simulink model "SWC_HALOUT_type"  (R2021b)
settings: Solver=FixedStepDiscrete  StartTime=0.0  StopTime=10.0  FixedStep=0.001  RelTol=1e-3
values from neighbouring files (symbols this model uses):
  DIDLen_APPPedalZP = uint16(3)    [vcu_local_hdr.m]
  DIDLen_APSFunConfig = uint16(16)    [vcu_local_hdr.m]
  DIDLen_AutoLock = uint16(1)    [vcu_local_hdr.m]
  DIDLen_AutoWipHSpdEN = uint16(1)    [vcu_local_hdr.m]
  DIDLen_DKCKey = uint16(8)    [vcu_local_hdr.m]
  DIDLen_DRLDis = uint16(1)    [vcu_local_hdr.m]
  DIDLen_DynoMode = uint16(1)    [vcu_local_hdr.m]
  DIDLen_FMHTimer = uint16(1)    [vcu_local_hdr.m]
  DIDLen_LFLowPresThre = uint16(1)    [vcu_local_hdr.m]
  DIDLen_LFSensorID = uint16(4)    [vcu_local_hdr.m]
  DIDLen_LRLowPresThre = uint16(1)    [vcu_local_hdr.m]
  DIDLen_LRSensorID = uint16(4)    [vcu_local_hdr.m]
  DIDLen_NVMPedalZP = uint16(3)    [vcu_local_hdr.m]
  DIDLen_RFLowPresThre = uint16(1)    [vcu_local_hdr.m]
  DIDLen_RFSensorID = uint16(4)    [vcu_local_hdr.m]
  DIDLen_RRLowPresThre = uint16(1)    [vcu_local_hdr.m]
  DIDLen_RRSensorID = uint16(4)    [vcu_local_hdr.m]
  DIDLen_SensorMode = uint16(1)    [vcu_local_hdr.m]
  DIDLen_TireSize = uint16(16)    [vcu_local_hdr.m]
  DIDLen_TPMSLearnSta = uint16(1)    [vcu_local_hdr.m]
  DIDLen_TurnLampFLThreCurr = uint16(1)    [vcu_local_hdr.m]
  DIDLen_TurnLampFRThreCurr = uint16(1)    [vcu_local_hdr.m]
  DIDLen_TurnLampRLThreCurr = uint16(1)    [vcu_local_hdr.m]
  DIDLen_TurnLampRRThreCurr = uint16(1)    [vcu_local_hdr.m]
  DIDLen_USSConfig = uint16(16)    [vcu_local_hdr.m]
  DIDLen_WhlPres = uint16(4)    [vcu_local_hdr.m]
  DIDLen_WhlSensorBattSta = uint16(1)    [vcu_local_hdr.m]
  DIDLen_WhlTmp = uint16(4)    [vcu_local_hdr.m]
  DIDLen_WipRLSCmdCutFilter = uint16(1)    [vcu_local_hdr.m]
  DIDLen_WipRLSCmdHoldFilter = uint16(1)    [vcu_local_hdr.m]
  DIDLen_XWDMode = uint16(1)    [vcu_local_hdr.m]
  DIDNum_APPPedalZP = uint16(0x0206)    [vcu_local_hdr.m]
  DIDNum_APSFunConfig = uint16(0x0903)    [vcu_local_hdr.m]
  DIDNum_AutoLock = uint16(0x0306)    [vcu_local_hdr.m]
  DIDNum_AutoWipHSpdEN = uint16(0x0308)    [vcu_local_hdr.m]
  DIDNum_DKCKey = uint16(0x0202)    [vcu_local_hdr.m]
  DIDNum_DRLDis = uint16(0x0307)    [vcu_local_hdr.m]
  DIDNum_DynoMode = uint16(0x0203)    [vcu_local_hdr.m]
  DIDNum_FMHTimer = uint16(0x0305)    [vcu_local_hdr.m]
  DIDNum_LFLowPresThre = uint16(0x0B08)    [vcu_local_hdr.m]
  DIDNum_LFSensorID = uint16(0x0B01)    [vcu_local_hdr.m]
  DIDNum_LRLowPresThre = uint16(0x0B0A)    [vcu_local_hdr.m]
  DIDNum_LRSensorID = uint16(0x0B03)    [vcu_local_hdr.m]
  DIDNum_NVMPedalZP = uint16(0x0207)    [vcu_local_hdr.m]
  DIDNum_RFLowPresThre = uint16(0x0B09)    [vcu_local_hdr.m]
  DIDNum_RFSensorID = uint16(0x0B02)    [vcu_local_hdr.m]
  DIDNum_RRLowPresThre = uint16(0x0B0B)    [vcu_local_hdr.m]
  DIDNum_RRSensorID = uint16(0x0B04)    [vcu_local_hdr.m]
  DIDNum_SensorMode = uint16(0x0B0C)    [vcu_local_hdr.m]
  DIDNum_TireSize = uint16(0x0902)    [vcu_local_hdr.m]
  DIDNum_TPMSLearnSta = uint16(0x0B0D)    [vcu_local_hdr.m]
  DIDNum_TurnLampFLThreCurr = uint16(0x0303)    [vcu_local_hdr.m]
  DIDNum_TurnLampFRThreCurr = uint16(0x0301)    [vcu_local_hdr.m]
  DIDNum_TurnLampRLThreCurr = uint16(0x0304)    [vcu_local_hdr.m]
  DIDNum_TurnLampRRThreCurr = uint16(0x0302)    [vcu_local_hdr.m]
  DIDNum_USSConfig = uint16(0x0901)    [vcu_local_hdr.m]
  DIDNum_WhlPres = uint16(0x0B05)    [vcu_local_hdr.m]
  DIDNum_WhlSensorBattSta = uint16(0x0B07)    [vcu_local_hdr.m]
  DIDNum_WhlTmp = uint16(0x0B06)    [vcu_local_hdr.m]
  DIDNum_WipRLSCmdCutFilter = uint16(0x030A)    [vcu_local_hdr.m]
  DIDNum_WipRLSCmdHoldFilter = uint16(0x0309)    [vcu_local_hdr.m]
  DIDNum_XWDMode = uint16(0x0201)    [vcu_local_hdr.m]
  ENUM_TPMSLearnStatus_LEARNED = uint8(  1  )    [vcu_local_hdr.m]
  ENUM_TPMSLearnStatus_LEARNFAIL = uint8(  2  )    [vcu_local_hdr.m]
  ENUM_TPMSLearnStatus_NOTLEARN = uint8(  0  )    [vcu_local_hdr.m]
  FALSE = boolean( 0 )    [vcu_local_hdr.m]    (also in vcu_local_hdrTA2.m)
  TRUE = boolean( 1 )    [vcu_local_hdr.m]    (also in vcu_local_hdrTA2.m)
  ZERO_INT = uint8(0)    [vcu_local_hdr.m]    (also in vcu_local_hdrTA2.m)
undefined symbols (not defined in the file or in its folder): f32_ApsOutVehSpdSig, R_DIDWriteCDD_CSOP_DIDSet_APPPedalZP, R_DIDWriteCDD_CSOP_DIDSet_APSFunConfig, R_DIDWriteCDD_CSOP_DIDSet_AutoLock, R_DIDWriteCDD_CSOP_DIDSet_AutoWipHSpdEN, R_DIDWriteCDD_CSOP_DIDSet_DKCKey, R_DIDWriteCDD_CSOP_DIDSet_DRLDis, R_DIDWriteCDD_CSOP_DIDSet_DynoMode, R_DIDWriteCDD_CSOP_DIDSet_FMHTimer, R_DIDWriteCDD_CSOP_DIDSet_LFLowPresThre, R_DIDWriteCDD_CSOP_DIDSet_LFSensorID, R_DIDWriteCDD_CSOP_DIDSet_LRLowPresThre, R_DIDWriteCDD_CSOP_DIDSet_LRSensorID, R_DIDWriteCDD_CSOP_DIDSet_NVMPedalZP, R_DIDWriteCDD_CSOP_DIDSet_RFLowPresThre, R_DIDWriteCDD_CSOP_DIDSet_RFSensorID, R_DIDWriteCDD_CSOP_DIDSet_RRLowPresThre, R_DIDWriteCDD_CSOP_DIDSet_RRSensorID, R_DIDWriteCDD_CSOP_DIDSet_SensorMode, R_DIDWriteCDD_CSOP_DIDSet_TireSize, R_DIDWriteCDD_CSOP_DIDSet_TPMSLearnSta, R_DIDWriteCDD_CSOP_DIDSet_TurnLampFLThreCurr, R_DIDWriteCDD_CSOP_DIDSet_TurnLampFRThreCurr, R_DIDWriteCDD_CSOP_DIDSet_TurnLampRLThreCurr, R_DIDWriteCDD_CSOP_DIDSet_TurnLampRRThreCurr, R_DIDWriteCDD_CSOP_DIDSet_USSConfig, R_DIDWriteCDD_CSOP_DIDSet_WhlPres, R_DIDWriteCDD_CSOP_DIDSet_WhlSensorBattSta, R_DIDWriteCDD_CSOP_DIDSet_WhlTmp, R_DIDWriteCDD_CSOP_DIDSet_WipRLSCmdCutFilter, R_DIDWriteCDD_CSOP_DIDSet_WipRLSCmdHoldFilter, R_DIDWriteCDD_CSOP_DIDSet_XWDMode, R_FDCCDD_Inner_CSOP_FDC_AppCallSleep, R_HALINCDD_CSOP_PAS_Handler, R_HALINCDD_CSOP_UDS_Main, R_HALOUT_APS_CSOP_ApsOutput, R_HALOUTCDD_CSOP_AppNmStateReq, R_HALOUTCDD_CSOP_ResetPedalZeroPosDone, R_HALOUTCDD_CSOP_SetAcoreRebootCmdACK, R_HALOUTCDD_CSOP_SetHazardIND, R_HALOUTCDD_CSOP_SetSysPwrStat, R_HALOUTCDD_CSOP_SleepRequest, R_HALOUTCDD_CSOP_TPMSSensorIDRegSetResults, R_IOExpOUT_CDD_CSOP_IOExpSetVal, R_J1939_CAN1_FD1_CE100_0_CSOP_Write_CAN1_FD1_CE100_0, R_J1939_CAN1_FD1_CE100_1_CSOP_Write_CAN1_FD1_CE100_1, R_NVMWriteCDD_Inner_NVM_WriteOperation, R_UDSCDD_CSOP_DdmRestartOperationCycle, R_WDGCDD_CSOP_Call_WDG_AppEnd, u16_DIDLen_APPPedalZP, u16_DIDLen_APSFunConfig, u16_DIDLen_AutoLock, u16_DIDLen_AutoWipHSpdEN, u16_DIDLen_DKCKey, u16_DIDLen_DRLDis, u16_DIDLen_DynoMode, u16_DIDLen_FMHTimer, u16_DIDLen_LFLowPresThre, u16_DIDLen_LFSensorID, u16_DIDLen_LRLowPresThre ... (+95)
libraries: FVT_lib x142, simulink x107, hdlsllib x6, hcu_lib x5, halout x1
(part 8 of 8)

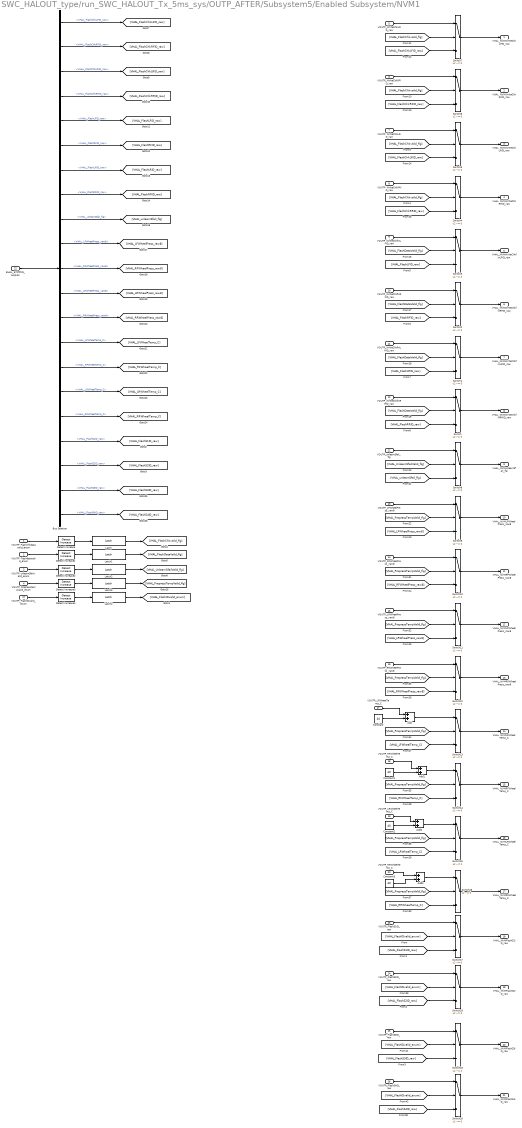
== system SWC_HALOUT_type/run_SWC_HALOUT_Tx_5ms_sys/OUTP_AFTER/Subsystem5/Enabled Subsystem/NVM1 ==
  VOUTP_Flashchkdatavalid_enum : Inport
  VOUTP_Flashdatavalid_enum : Inport  Port=2
  VOUTP_unlearnSfailvalid_enum : Inport  Port=3
  VOUTP_Prepresstempvalid_enum : Inport  Port=4
  VOUTP_WriteChkLFID_raw : Inport  Port=5
  VOUTP_WriteChkRFID_raw : Inport  Port=6
  VOUTP_WriteChkLRID_raw : Inport  Port=7
  VOUTP_WriteChkRRID_raw : Inport  Port=8
  VOUTP_WriteChkfinLFID_raw : Inport  Port=9
  VOUTP_WriteChkfinRFID_raw : Inport  Port=10
  VOUTP_WriteChkfinLRID_raw : Inport  Port=11
  VOUTP_WriteChkfinRRID_raw : Inport  Port=12
  VOUTP_LFWheelPress_raw8 : Inport  Port=13
  VOUTP_RFWheelPress_raw8 : Inport  Port=14
  VOUTP_LRWheelPress_raw8 : Inport  Port=15
  VOUTP_RRWheelPress_raw8 : Inport  Port=16
  VOUTP_LFWheelTemp_C : Inport  Port=17
  VOUTP_RFWheelTemp_C : Inport  Port=18
  VOUTP_LRWheelTemp_C : Inport  Port=19
  VOUTP_RRWheelTemp_C : Inport  Port=20
  VOUTP_unlearnSfali_flg : Inport  Port=21
  BHAL_SYSTPMS_outputs : Inport  Port=22
  VOUTP_FlashS1ID_raw : Inport  Port=23
  VOUTP_FlashS2ID_raw : Inport  Port=24
  VOUTP_FlashS3ID_raw : Inport  Port=25
  VOUTP_FlashS4ID_raw : Inport  Port=26
  VOUTP_FlashIDvalid_enum : Inport  Port=27
  Add{,1..3} (4 alike) : Sum
  Bus Selector : BusSelector  OutputSignals=VHAL_FlashChkLFID_raw,VHAL_FlashChkRFID_raw,VHAL_FlashChkLRID_raw,VHAL_FlashChkRRID_raw,VHAL_FlashLFID_raw,VHAL_FlashRFID_raw,VHAL_FlashLRID_raw,VHAL_FlashRRID_raw,VHAL_unlearnSfali_flg,VHAL_LFWheelPress_raw8,VHAL_RFWheelPress_raw8,VHAL_LRWheelPress_raw8,VHAL_RRWheelPress_raw8,VHAL_LFWheelTemp_C,VHAL_RFWheelTemp_C,VHAL_LRWheelTemp_C,VHAL_RRWheelTemp_C,VHAL_FlashS1ID_raw,VHAL_FlashS2ID_raw,VHAL_FlashS3ID_raw,VHAL_FlashS4ID_raw
  Constant{,1..3} (4 alike) : Constant  Value=40
  Detect Increase{,1..4} (5 alike) : simulink/Logic and Bit Operations/Detect Increase  vinit=0.0  OutDataTypeStr=boolean
  Latch{,1..4} (5 alike) : hcu_lib/Basic_Blocks/Latch
  Switch{,1..20} (21 alike) : Switch  Criteria=u2 ~= 0
  VHAL_NVMWriteChkLFID_raw : Outport
  VHAL_NVMWriteChkRFID_raw : Outport  Port=2
  VHAL_NVMWriteChkLRID_raw : Outport  Port=3
  VHAL_NVMWriteChkRRID_raw : Outport  Port=4
  VHAL_NVMWriteChkfinLFID_raw : Outport  Port=5
  VHAL_NVMWriteChkfinRFID_raw : Outport  Port=6
  VHAL_NVMWriteChkfinLRID_raw : Outport  Port=7
  VHAL_NVMWriteChkfinRRID_raw : Outport  Port=8
  VHAL_NVMunlearnSfali_flg : Outport  Port=9
  VHAL_NVMLFWheelPress_raw8 : Outport  Port=10
  VHAL_NVMRFWheelPress_raw8 : Outport  Port=11
  VHAL_NVMLRWheelPress_raw8 : Outport  Port=12
  VHAL_NVMRRWheelPress_raw8 : Outport  Port=13
  VHAL_NVMLFWheelTemp_C : Outport  Port=14
  VHAL_NVMRFWheelTemp_C : Outport  Port=15
  VHAL_NVMLRWheelTemp_C : Outport  Port=16
  VHAL_NVMRRWheelTemp_C : Outport  Port=17
  VHAL_NVMFlashS1ID_raw : Outport  Port=18
  VHAL_NVMFlashS2ID_raw : Outport  Port=19
  VHAL_NVMFlashS3ID_raw : Outport  Port=20
  VHAL_NVMFlashS4ID_raw : Outport  Port=21
  wires:
  Bus Selector/2 -> [VHAL_FlashChkRFID_raw]  "<VHAL_FlashChkRFID_raw>"
  Bus Selector/1 -> [VHAL_FlashChkLFID_raw]  "<VHAL_FlashChkLFID_raw>"
  Bus Selector/11 -> [VHAL_RFWheelPress_raw8]  "<VHAL_RFWheelPress_raw8>"
  Bus Selector/3 -> [VHAL_FlashChkLRID_raw]  "<VHAL_FlashChkLRID_raw>"
  Bus Selector/7 -> [VHAL_FlashLRID_raw]  "<VHAL_FlashLRID_raw>"
  Bus Selector/5 -> [VHAL_FlashLFID_raw]  "<VHAL_FlashLFID_raw>"
  Bus Selector/6 -> [VHAL_FlashRFID_raw]  "<VHAL_FlashRFID_raw>"
  Bus Selector/8 -> [VHAL_FlashRRID_raw]  "<VHAL_FlashRRID_raw>"
  Bus Selector/14 -> [VHAL_LFWheelTemp_C]  "<VHAL_LFWheelTemp_C>"
  Bus Selector/9 -> [VHAL_unlearnSfali_flg]  "<VHAL_unlearnSfali_flg>"
  Bus Selector/13 -> [VHAL_RRWheelPress_raw8]  "<VHAL_RRWheelPress_raw8>"
  Bus Selector/4 -> [VHAL_FlashChkRRID_raw]  "<VHAL_FlashChkRRID_raw>"
  Bus Selector/12 -> [VHAL_LRWheelPress_raw8]  "<VHAL_LRWheelPress_raw8>"
  BHAL_SYSTPMS_outputs/1 -> Bus Selector/1
  Bus Selector/15 -> [VHAL_RFWheelTemp_C]  "<VHAL_RFWheelTemp_C>"
  Bus Selector/10 -> [VHAL_LFWheelPress_raw8]  "<VHAL_LFWheelPress_raw8>"
  Bus Selector/17 -> [VHAL_RRWheelTemp_C]  "<VHAL_RRWheelTemp_C>"
  Bus Selector/16 -> [VHAL_LRWheelTemp_C]  "<VHAL_LRWheelTemp_C>"
  Switch/1 -> VHAL_NVMWriteChkfinRRID_raw/1
  Switch1/1 -> VHAL_NVMWriteChkfinLRID_raw/1
  Switch2/1 -> VHAL_NVMWriteChkfinRFID_raw/1
  Switch3/1 -> VHAL_NVMWriteChkfinLFID_raw/1
  Switch4/1 -> VHAL_NVMWriteChkRRID_raw/1
  Switch5/1 -> VHAL_NVMWriteChkLRID_raw/1
  Switch6/1 -> VHAL_NVMWriteChkRFID_raw/1
  Switch7/1 -> VHAL_NVMWriteChkLFID_raw/1
  Switch8/1 -> VHAL_NVMunlearnSfali_flg/1
  VOUTP_WriteChkRFID_raw/1 -> Switch6/1
  VOUTP_WriteChkLFID_raw/1 -> Switch7/1
  VOUTP_WriteChkfinLFID_raw/1 -> Switch3/1
  VOUTP_WriteChkRRID_raw/1 -> Switch4/1
  VOUTP_WriteChkLRID_raw/1 -> Switch5/1
  VOUTP_WriteChkfinRRID_raw/1 -> Switch/1
  VOUTP_WriteChkfinLRID_raw/1 -> Switch1/1
  [VHAL_FlashRRID_raw] -> Switch/3
  VOUTP_WriteChkfinRFID_raw/1 -> Switch2/1
  [VHAL_FlashChkvalid_flg] -> Switch7/2
  [VHAL_FlashChkvalid_flg] -> Switch4/2
  [VHAL_FlashRFID_raw] -> Switch2/3
  [VHAL_FlashLFID_raw] -> Switch3/3
  [VHAL_FlashChkLFID_raw] -> Switch7/3
  [VHAL_FlashChkLRID_raw] -> Switch5/3
  [VHAL_FlashDataValid_flg] -> Switch1/2
  [VHAL_FlashChkRRID_raw] -> Switch4/3
  [VHAL_FlashDataValid_flg] -> Switch/2
  [VHAL_FlashDataValid_flg] -> Switch3/2
  [VHAL_FlashChkvalid_flg] -> Switch5/2
  [VHAL_FlashDataValid_flg] -> Switch2/2
  [VHAL_FlashChkRFID_raw] -> Switch6/3
  [VHAL_FlashLRID_raw] -> Switch1/3
  [VHAL_FlashChkvalid_flg] -> Switch6/2
  VOUTP_Prepresstempvalid_enum/1 -> Detect Increase3/1
  VOUTP_unlearnSfailvalid_enum/1 -> Detect Increase2/1
  VOUTP_Flashdatavalid_enum/1 -> Detect Increase1/1
  VOUTP_Flashchkdatavalid_enum/1 -> Detect Increase/1
  Latch3/1 -> [VHAL_PrepressTempValid_flg]
  Detect Increase/1 -> Latch/1
  Detect Increase2/1 -> Latch2/1
  Latch1/1 -> [VHAL_FlashDataValid_flg]
  Latch2/1 -> [VHAL_UnlearnSfailValid_flg]
  Latch/1 -> [VHAL_FlashChkvalid_flg]
  Detect Increase3/1 -> Latch3/1
  Detect Increase1/1 -> Latch1/1
  [VHAL_unlearnSfali_flg] -> Switch8/3
  VOUTP_unlearnSfali_flg/1 -> Switch8/1
  [VHAL_UnlearnSfailValid_flg] -> Switch8/2
  VOUTP_RRWheelTemp_C/1 -> Add3/1
  VOUTP_LFWheelTemp_C/1 -> Add/1
  VOUTP_RFWheelTemp_C/1 -> Add1/1
  VOUTP_LRWheelTemp_C/1 -> Add2/1
  VOUTP_LFWheelPress_raw8/1 -> Switch9/1
  Switch16/1 -> VHAL_NVMRRWheelTemp_C/1
  Switch13/1 -> VHAL_NVMLFWheelTemp_C/1
  [VHAL_LRWheelTemp_C] -> Switch15/3
  Switch15/1 -> VHAL_NVMLRWheelTemp_C/1
  Switch14/1 -> VHAL_NVMRFWheelTemp_C/1
  [VHAL_PrepressTempValid_flg] -> Switch16/2
  VOUTP_RFWheelPress_raw8/1 -> Switch10/1
  Switch9/1 -> VHAL_NVMLFWheelPress_raw8/1
  Switch10/1 -> VHAL_NVMRFWheelPress_raw8/1
  [VHAL_LFWheelTemp_C] -> Switch13/3
  Switch11/1 -> VHAL_NVMLRWheelPress_raw8/1
  [VHAL_PrepressTempValid_flg] -> Switch9/2
  [VHAL_RFWheelTemp_C] -> Switch14/3
  [VHAL_RRWheelPress_raw8] -> Switch12/3
  Switch12/1 -> VHAL_NVMRRWheelPress_raw8/1
  [VHAL_PrepressTempValid_flg] -> Switch12/2
  [VHAL_PrepressTempValid_flg] -> Switch14/2
  [VHAL_LFWheelPress_raw8] -> Switch9/3
  [VHAL_LRWheelPress_raw8] -> Switch11/3
  [VHAL_RFWheelPress_raw8] -> Switch10/3
  [VHAL_PrepressTempValid_flg] -> Switch15/2
  VOUTP_LRWheelPress_raw8/1 -> Switch11/1
  [VHAL_PrepressTempValid_flg] -> Switch10/2
  [VHAL_RRWheelTemp_C] -> Switch16/3
  [VHAL_PrepressTempValid_flg] -> Switch13/2
  [VHAL_PrepressTempValid_flg] -> Switch11/2
  VOUTP_RRWheelPress_raw8/1 -> Switch12/1
  Detect Increase4/1 -> Latch4/1
  Latch4/1 -> [VHAL_FlashIDvalid_enum]
  VOUTP_FlashIDvalid_enum/1 -> Detect Increase4/1
  [VHAL_FlashS1ID_raw] -> Switch17/3
  [VHAL_FlashIDvalid_enum] -> Switch17/2
  Switch17/1 -> VHAL_NVMFlashS1ID_raw/1
  VOUTP_FlashS1ID_raw/1 -> Switch17/1
  Bus Selector/18 -> [VHAL_FlashS1ID_raw]  "<VHAL_FlashS1ID_raw>"
  Bus Selector/19 -> [VHAL_FlashS2ID_raw]  "<VHAL_FlashS2ID_raw>"
  Bus Selector/20 -> [VHAL_FlashS3ID_raw]  "<VHAL_FlashS3ID_raw>"
  Bus Selector/21 -> [VHAL_FlashS4ID_raw]  "<VHAL_FlashS4ID_raw>"
  [VHAL_FlashS2ID_raw] -> Switch18/3
  Switch18/1 -> VHAL_NVMFlashS2ID_raw/1
  VOUTP_FlashS2ID_raw/1 -> Switch18/1
  [VHAL_FlashIDvalid_enum] -> Switch18/2
  Switch19/1 -> VHAL_NVMFlashS3ID_raw/1
  [VHAL_FlashS3ID_raw] -> Switch19/3
  [VHAL_FlashIDvalid_enum] -> Switch19/2
  VOUTP_FlashS3ID_raw/1 -> Switch19/1
  Switch20/1 -> VHAL_NVMFlashS4ID_raw/1
  [VHAL_FlashS4ID_raw] -> Switch20/3
  [VHAL_FlashIDvalid_enum] -> Switch20/2
  VOUTP_FlashS4ID_raw/1 -> Switch20/1
  Constant/1 -> Add/2
  Add/1 -> Switch13/1
  Add1/1 -> Switch14/1
  Constant1/1 -> Add1/2
  Add2/1 -> Switch15/1
  Constant2/1 -> Add2/2
  Add3/1 -> Switch16/1
  Constant3/1 -> Add3/2

== system SWC_HALOUT_type/run_SWC_HALOUT_Tx_5ms_sys/OUTP_AFTER/Subsystem5/Enabled Subsystem/Subsystem ==
  VOUTP_DiagFMHT_s : Inport
  Add1 : Sum  Inputs=+-
  Constant45 : Constant  Value=10
  Gain4 : Gain  Gain=1/5
  Saturation : Saturate  UpperLimit=150  LowerLimit=5
  Out1 : Outport
  wires:
  VOUTP_DiagFMHT_s/1 -> Add1/1
  Constant45/1 -> Add1/2
  Gain4/1 -> Out1/1
  Saturation/1 -> Gain4/1
  Add1/1 -> Saturation/1

== stateflow chart SWC_HALOUT_type/run_SWC_HALOUT_Tx_5ms_sys/hcu_main_sched ==
  state Main_Scheduler
    (default) -> (junction 31) : {
        |   Sys_Init_done = FALSE;
        |   trig_Read_NVM_00;
        |   trig_ReadIMUOffset_00;
        | }
    Main_Scheduler -> (junction 31) : {Sys_Init_done = TRUE;}
    (junction 31) -> (junction 34) [order 1] : [
        |    Sys_Init_done &&...
        |    !VHAL_FusionSchedReq_flg
        | ]
    (junction 31) -> (junction 38) [order 2]
    (junction 34) -> (junction 36) : {
        |     trig_WDG;
        |     trig_GetNMID;
        |     trig_GetDID;
        |     trig_HAL_IN_10;
        |     trig_HAL_CDD_10_1;
        |     trig_HAL_DKC_10_2;
        |     trig_HAL_DKC_10_3;
        |     trig_INP_20;
        |     trig_APP_30;
        |     trig_OUTP_40;
        |     trig_OUTP_AFTER_40_1;
        |     trig_SetDID;
        |     trig_HAL_OUT_50;
        |     trig_HAL_OUTAFTER_50_1;
        |    }
    (junction 36) -> (junction 38)
  (default) -> Main_Scheduler
  data: VHAL_FusionSchedReq_flg input; Sys_Init_done local double; FALSE parameter; TRUE parameter
  events: trig_Read_NVM_00 output FUNCTION_CALL_EVENT; trig_ReadIMUOffset_00 output FUNCTION_CALL_EVENT; trig_WDG output FUNCTION_CALL_EVENT; trig_GetNMID output FUNCTION_CALL_EVENT; trig_GetDID output FUNCTION_CALL_EVENT; trig_HAL_IN_10 output FUNCTION_CALL_EVENT; trig_HAL_CDD_10_1 output FUNCTION_CALL_EVENT; trig_HAL_DKC_10_2 output FUNCTION_CALL_EVENT; trig_HAL_DKC_10_3 output FUNCTION_CALL_EVENT; trig_INP_20 output FUNCTION_CALL_EVENT; trig_APP_30 output FUNCTION_CALL_EVENT; trig_OUTP_40 output FUNCTION_CALL_EVENT; trig_OUTP_AFTER_40_1 output FUNCTION_CALL_EVENT; trig_SetDID output FUNCTION_CALL_EVENT; trig_HAL_OUT_50 output FUNCTION_CALL_EVENT; trig_HAL_OUTAFTER_50_1 output FUNCTION_CALL_EVENT
